simulink model "Sensor"  (R2024b)
settings: Solver=VariableStepAuto  StartTime=0  StopTime=12  RelTol=1e-3
undefined symbols (not defined in the file or in its folder): Defined, driving, Ego, Lane, simStepSize, User
libraries: roadrunnerscenario x7, drivingscenarioandsensors x1
settings Model: Creator=andre  LastModifiedBy=andre

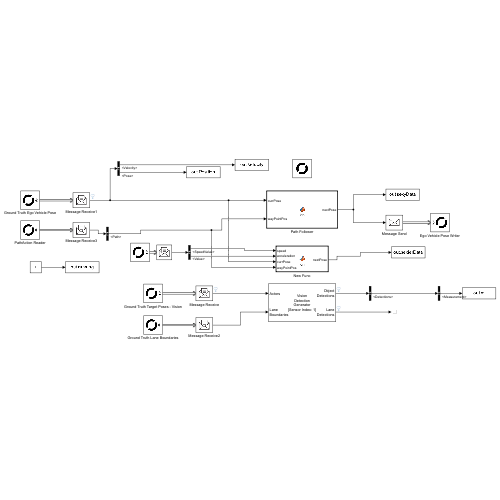
[thumbnail: Simulink's stored preview of the top-level diagram]
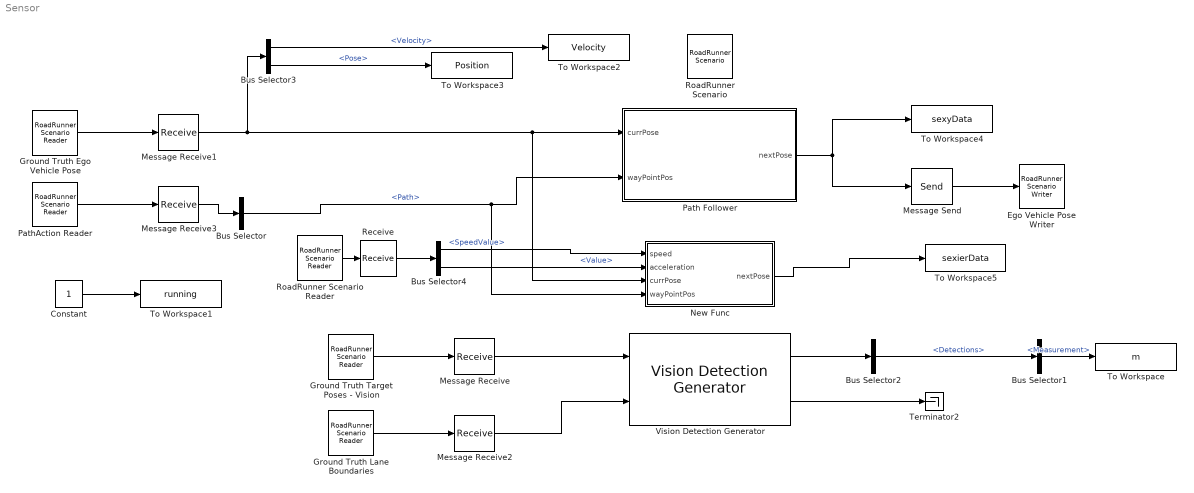
== system Sensor ==
  Bus Selector : BusSelector  OutputSignals=PathTarget.Path
  Bus Selector1 : BusSelector  OutputSignals=Measurement
  Bus Selector2 : BusSelector  OutputSignals=Detections
  Bus Selector3 : BusSelector  OutputSignals=Velocity,Pose
  Bus Selector4 : BusSelector  OutputSignals=SpeedTarget.SpeedValue,TransitionDynamics.Value
  Constant : Constant
  Ego Vehicle Pose Writer : roadrunnerscenario/RoadRunner Scenario Writer  TopicCategory=Actor  ActorCategory=All Types  EventType=Action Complete  UserDefinedEvent=Event1  VehicleType=Vehicle Pose  TopicType=Actor Pose
  Ground Truth Ego Vehicle Pose : roadrunnerscenario/RoadRunner Scenario Reader  TopicCategory=Actor  ActorCategory=All Types  ActionType=Path Following  EventType=User-Defined  TopicType=Actor Pose  VehicleType=Vehicle Pose  UserDefinedAction=Action1  UserDefinedEvent=Event1  Filter=Self  SensorTopic=Target Poses  LaneBoundaryOutputTopic=Ego-Lane  SensorID=1  SampleTime=simStepSize
  Ground Truth Lane Boundaries : roadrunnerscenario/RoadRunner Scenario Reader  TopicCategory=Sensor  ActorCategory=All Types  ActionType=Path Following  EventType=User-Defined  TopicType=Actor Pose  VehicleType=Vehicle Pose  UserDefinedAction=Action1  UserDefinedEvent=Event1  Filter=Self  SensorTopic=Lane Boundaries  LaneBoundaryOutputTopic=Ego and Adjacent Lanes  SensorID=1  SampleTime=simStepSize
  Ground Truth Target Poses - Vision : roadrunnerscenario/RoadRunner Scenario Reader  TopicCategory=Sensor  ActorCategory=All Types  ActionType=Path Following  EventType=User-Defined  TopicType=Actor Specifications  VehicleType=Vehicle Specifications  UserDefinedAction=Action1  UserDefinedEvent=Event1  Filter=Self  SensorTopic=Target Poses  LaneBoundaryOutputTopic=Ego-Lane  SensorID=1  SampleTime=simStepSize
  Message Receive{,1..3} (4 alike) : Receive  InputPortMessageModes=m  UseInternalQueue=off  SampleTime=simStepSize
  Message Send : Send  OutputPortMessageModes=m
  New Func : MATLAB Function  TreatAsAtomicUnit=on
  Path Follower : MATLAB Function  TreatAsAtomicUnit=on
  PathAction Reader : roadrunnerscenario/RoadRunner Scenario Reader  TopicCategory=Action  ActorCategory=All Types  ActionType=Path Following  EventType=User-Defined  TopicType=Actor Specifications  VehicleType=Vehicle Specifications  UserDefinedAction=Action1  UserDefinedEvent=Event1  Filter=Self  SensorTopic=Target Poses  LaneBoundaryOutputTopic=Ego-Lane  SensorID=1  SampleTime=simStepSize
  Receive : Receive  InputPortMessageModes=m  UseInternalQueue=off  QueueOverwriting=on  QueueLength=1  QueueType=LIFO
  RoadRunner Scenario : roadrunnerscenario/RoadRunner Scenario  UserDefinedActions={}  UserDefinedEvents={}
  RoadRunner Scenario Reader : roadrunnerscenario/RoadRunner Scenario Reader  TopicCategory=Action  ActorCategory=All Types  ActionType=Speed Change  EventType=User-Defined  TopicType=Actor Specifications  VehicleType=Vehicle Specifications  UserDefinedAction=Action1  UserDefinedEvent=Event1  Filter=Self  SensorTopic=Target Poses  LaneBoundaryOutputTopic=Ego-Lane  SensorID=1  SampleTime=0
  Terminator2 : Terminator
  To Workspace : ToWorkspace  VariableName=m  SampleTime=-1
  To Workspace1 : ToWorkspace  VariableName=running  SaveFormat=Timeseries  SampleTime=-1
  To Workspace2 : ToWorkspace  VariableName=Velocity  SaveFormat=Timeseries  SampleTime=-1
  To Workspace3 : ToWorkspace  VariableName=Position  SaveFormat=Timeseries  SampleTime=-1
  To Workspace4 : ToWorkspace  VariableName=sexyData  SaveFormat=Timeseries  SampleTime=-1
  To Workspace5 : ToWorkspace  VariableName=sexierData  SaveFormat=Timeseries  SampleTime=-1
  Vision Detection Generator : drivingscenarioandsensors/Vision Detection Generator  SensorIndex=1  DetectorOutput=Lanes and objects  UpdateInterval=simStepSize  LaneUpdateInterval=simStepSize  SensorLocation=[1.2 0]  Height=1.1  Yaw=0  Pitch=1  Roll=0  BusNameSource=Auto  BusName=BusObjectDetections  BusName2Source=Auto  BusName2=BusLaneDetections  MaxNumDetectionsSource=Property  MaxNumDetections=1  MaxNumLanesSource=Property  MaxNumLanes=30  DetectionCoordinates=Ego Cartesian  SimulateUsing=Interpreted execution  MaxRange=150  BoundingBoxAccuracy=5  ProcessNoiseIntensity=5  MaxSpeed=100  MaxAllowedOcclusion=0.5  MinObjectImageSize=[ 15, 15 ]  DetectionProbability=1  FalsePositivesPerImage=0  MinLaneImageSize=[ 20, 3 ]  LaneBoundaryAccuracy=3  HasNoise=off  InitialSeedSource=Repeatable  InitialSeed=0  UsedSeed=driving.internal.SimulinkUtilities.seedManager(gcb)  ActorProfilesSource=From Scenario Reader block  ActorProfilesParameters=driving.internal.ActorProfilesParameters  ActorProfilesExpression=actorProfiles  Intrinsics=driving.internal.cameraIntrinsics('FocalLength',[ 1200, 1200 ])
  wires:
  Message Receive1/1 -> Bus Selector3/1, New Func/3(currPose), Path Follower/1(currPose)
  New Func/1(nextPose) -> To Workspace5/1
  Path Follower/1(nextPose) -> To Workspace4/1, Message Send/1
  Message Receive3/1 -> Bus Selector/1
  Vision Detection Generator/1 -> Bus Selector2/1
  Message Receive2/1 -> Vision Detection Generator/2
  PathAction Reader/1 -> Message Receive3/1
  Bus Selector2/1 -> Bus Selector1/1  "<Detections>"
  Constant/1 -> To Workspace1/1
  Ground Truth Ego Vehicle Pose/1 -> Message Receive1/1
  Bus Selector3/1 -> To Workspace2/1  "<Velocity>"
  Message Receive/1 -> Vision Detection Generator/1
  Bus Selector4/2 -> New Func/2(acceleration)  "<Value>"
  Receive/1 -> Bus Selector4/1
  Ground Truth Target Poses - Vision/1 -> Message Receive/1
  RoadRunner Scenario Reader/1 -> Receive/1
  Bus Selector1/1 -> To Workspace/1  "<Measurement>"
  Vision Detection Generator/2 -> Terminator2/1
  Message Send/1 -> Ego Vehicle Pose Writer/1
  Bus Selector/1 -> New Func/4(wayPointPos), Path Follower/2(wayPointPos)  "<Path>"
  Ground Truth Lane Boundaries/1 -> Message Receive2/1
  Bus Selector3/2 -> To Workspace3/1  "<Pose>"
  Bus Selector4/1 -> New Func/1(speed)  "<SpeedValue>"

== matlab function Sensor/New Func ==
  data: speed input; nextPose output; acceleration input; simStepSize parameter; currPose input; wayPointPos input
function nextPose = fcn(speed,acceleration,simStepSize,currPose, wayPointPos)

currSpeed=sqrt((currPose.Velocity(1)^2)+(currPose.Velocity(2)^2)+(currPose.Velocity(3)^2));

sign=1;
if currSpeed>speed
    sign=-1;
end

egoSpeed=speed+sign*acceleration*simStepSize;


% Declare persistent variables for simulation and retain only non zero
% elements in the array of waypoints 
persistent wayPointIdx wayPointPosInterp headingAnglesInterp numWayPoints
wayPointPos = reshape(wayPointPos(wayPointPos~=0),[],2);

% Extract poses for the entire path before simulation begins
if isempty(wayPointIdx)
    
    wayPointIdx = 2;

    % Pre-allocate arrays
    numInputPoints = length(wayPointPos);
    trueTimes = zeros(numInputPoints+1,1);
    headingAngles = zeros(numInputPoints,1);
    wayPointPosInterp = [];
    headingAnglesInterp = [];

    startPoint = [currPose.Pose(1,4) currPose.Pose(2,4)];
    currPoint = startPoint;

    % Loop through all the input points
    for i=1:numInputPoints

        % Calculate distance from the current point to the next point
        nextPoint = wayPointPos(i,1:2);
        delXY = nextPoint-currPoint;
        absDistToNextPoint = norm(delXY);
        
        % Calculate time of arrival at the next wayPoint based on the
        % set constant speed. Alternatively, you can set the timing profile
        % in RoadRunner for waypoints and use those here 
        trueTimes(i+1) = absDistToNextPoint/egoSpeed + trueTimes(i);
        
        % Calculate the heading angle to proceed towards the next waypoint
        headingAngles(i) = atan2d(delXY(2),delXY(1))-90;
        
        % Based on the simulation step size, calculate the time vector
        % between arrival times at previous waypoint and the current waypoint
        tvec = trueTimes(i):simStepSize:trueTimes(i+1);
        
        % Interpolate X and Y positions between the current and next waypoints
        % along the entire time vector. Store them
        interpPosPointsX = interp1(linspace(trueTimes(i),trueTimes(i+1),100),...
                linspace(currPoint(1),nextPoint(1),100),...
                tvec)';
    
        interpPosPointsY = interp1(linspace(trueTimes(i),trueTimes(i+1),100),...
                linspace(currPoint(2),nextPoint(2),100),...
                tvec)';
        
        wayPointPosInterp = [wayPointPosInterp;[interpPosPointsX interpPosPointsY]];

        % Use the constant heading angle towards the next waypoint for all
        % interpolated points between them
        headingAnglesInterp = [headingAnglesInterp;headingAngles(i)*ones(size(interpPosPointsX))];

        currPoint = nextPoint;
    end

    % Get the new total number of waypoints after interpolation
    numWayPoints = length(wayPointPosInterp);
end

% At each time step of the simulation, send the next waypoint position from the
% interpolated waypoint array until ego vehicle arrives at the last waypoint
nextPose = currPose;
class(nextPose)
nextPose.Pose(1,4) = wayPointPosInterp(wayPointIdx,1);
nextPose.Pose(2,4) = wayPointPosInterp(wayPointIdx,2);

% Convert the heading angle (yaw) to a rotation matrix
nextPose.Pose(1:3,1:3) = [cosd(headingAnglesInterp(wayPointIdx)) -sind(headingAnglesInterp(wayPointIdx)) 0;...
                          sind(headingAnglesInterp(wayPointIdx)) cosd(headingAnglesInterp(wayPointIdx)) 0;...
                          0 0 1];

if(wayPointIdx<numWayPoints)
    wayPointIdx = wayPointIdx + 1;
end

end

== matlab function Sensor/Path Follower ==
  data: currPose input; wayPointPos input; nextPose output Bus: BusActorRuntime; simStepSize parameter
function nextPose  = fcn(currPose, wayPointPos,simStepSize)

% Set ego vehicle speed
egoSpeed  = 18;

% Declare persistent variables for simulation and retain only non zero
% elements in the array of waypoints 
persistent wayPointIdx wayPointPosInterp headingAnglesInterp numWayPoints
wayPointPos = reshape(wayPointPos(wayPointPos~=0),[],2);

% Extract poses for the entire path before simulation begins
if isempty(wayPointIdx)
    
    wayPointIdx = 2;

    % Pre-allocate arrays
    numInputPoints = length(wayPointPos);
    trueTimes = zeros(numInputPoints+1,1);
    headingAngles = zeros(numInputPoints,1);
    wayPointPosInterp = [];
    headingAnglesInterp = [];

    startPoint = [currPose.Pose(1,4) currPose.Pose(2,4)];
    currPoint = startPoint;

    % Loop through all the input points
    for i=1:numInputPoints

        % Calculate distance from the current point to the next point
        nextPoint = wayPointPos(i,1:2);
        delXY = nextPoint-currPoint;
        absDistToNextPoint = norm(delXY);
        
        % Calculate time of arrival at the next wayPoint based on the
        % set constant speed. Alternatively, you can set the timing profile
        % in RoadRunner for waypoints and use those here 
        trueTimes(i+1) = absDistToNextPoint/egoSpeed + trueTimes(i);
        
        % Calculate the heading angle to proceed towards the next waypoint
        headingAngles(i) = atan2d(delXY(2),delXY(1))-90;
        
        % Based on the simulation step size, calculate the time vector
        % between arrival times at previous waypoint and the current waypoint
        tvec = trueTimes(i):simStepSize:trueTimes(i+1);
        
        % Interpolate X and Y positions between the current and next waypoints
        % along the entire time vector. Store them
        interpPosPointsX = interp1(linspace(trueTimes(i),trueTimes(i+1),100),...
                linspace(currPoint(1),nextPoint(1),100),...
                tvec)';
    
        interpPosPointsY = interp1(linspace(trueTimes(i),trueTimes(i+1),100),...
                linspace(currPoint(2),nextPoint(2),100),...
                tvec)';
        
        wayPointPosInterp = [wayPointPosInterp;[interpPosPointsX interpPosPointsY]];

        % Use the constant heading angle towards the next waypoint for all
        % interpolated points between them
        headingAnglesInterp = [headingAnglesInterp;headingAngles(i)*ones(size(interpPosPointsX))];

        currPoint = nextPoint;
    end

    % Get the new total number of waypoints after interpolation
    numWayPoints = length(wayPointPosInterp);
end

% At each time step of the simulation, send the next waypoint position from the
% interpolated waypoint array until ego vehicle arrives at the last waypoint
nextPose = currPose;
nextPose.Pose(1,4) = wayPointPosInterp(wayPointIdx,1);
nextPose.Pose(2,4) = wayPointPosInterp(wayPointIdx,2);

% Convert the heading angle (yaw) to a rotation matrix
nextPose.Pose(1:3,1:3) = [cosd(headingAnglesInterp(wayPointIdx)) -sind(headingAnglesInterp(wayPointIdx)) 0;...
                          sind(headingAnglesInterp(wayPointIdx)) cosd(headingAnglesInterp(wayPointIdx)) 0;...
                          0 0 1];

if(wayPointIdx<numWayPoints)
    wayPointIdx = wayPointIdx + 1;
end

end
